simulink model "ratelimiting_test"  (R2021a)
settings: Solver=FixedStepAuto  StartTime=0.0  StopTime=25  FixedStep=0.01  RelTol=1e-3
settings Model: Creator=loren  LastModifiedBy=loren

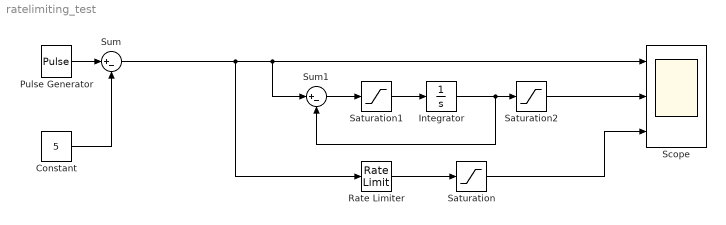
== system ratelimiting_test ==
  Constant : Constant  Value=5
  Integrator : Integrator
  Pulse Generator : DiscretePulseGenerator  PulseType=Time based  Amplitude=10  Period=10  PulseWidth=50
  Rate Limiter : RateLimiter  RisingSlewLimit=5  FallingSlewLimit=-5  SampleTimeMode=inherited
  Saturation : Saturate  UpperLimit=4  LowerLimit=-4
  Saturation1 : Saturate  UpperLimit=4  LowerLimit=-4
  Saturation2 : Saturate  UpperLimit=4  LowerLimit=-4
  Scope : Scope  NumInputPorts=3
  Sum : Sum  Inputs=|+-
  Sum1 : Sum  Inputs=|+-
  wires:
  Sum/1 -> Rate Limiter/1, Sum1/1, Scope/1
  Rate Limiter/1 -> Saturation/1
  Saturation/1 -> Scope/3
  Pulse Generator/1 -> Sum/1
  Constant/1 -> Sum/2
  Sum1/1 -> Saturation1/1
  Saturation1/1 -> Integrator/1
  Integrator/1 -> Saturation2/1, Sum1/2
  Saturation2/1 -> Scope/2
